simulink model "t3"  (R2016a)
settings: Solver=VariableStepAuto  StartTime=0.0  StopTime=10.0  RelTol=1e-3
settings Model: Creator=admin  LastModifiedBy=admin

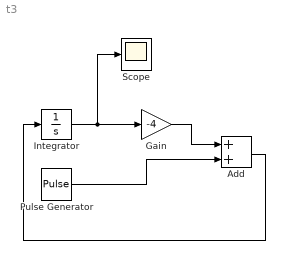
== system t3 ==
  Add : Sum
  Gain : Gain  Gain=-4
  Integrator : Integrator
  Pulse Generator : DiscretePulseGenerator  PulseType=Time based  Period=10  PulseWidth=5
  Scope : Scope
  wires:
  Integrator/1 -> Scope/1, Gain/1
  Gain/1 -> Add/1
  Pulse Generator/1 -> Add/2
  Add/1 -> Integrator/1
